simulink model "SLtest"  (R2024b)
settings: Solver=VariableStepAuto  StartTime=0.0  StopTime=10.0  RelTol=1e-3
settings Model: Creator=lazar  LastModifiedBy=lazar

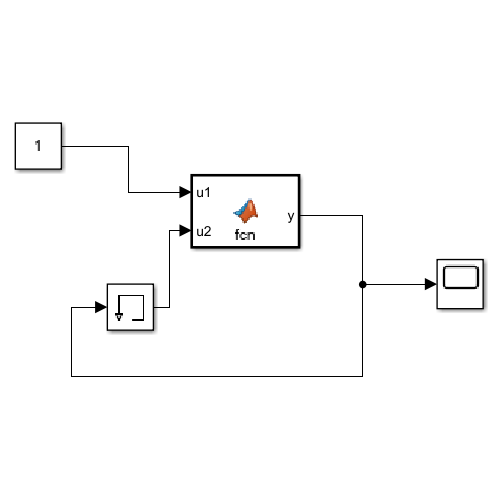
[thumbnail: Simulink's stored preview of the top-level diagram]
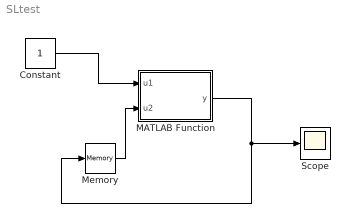
== system SLtest ==
  Constant : Constant
  MATLAB Function : MATLAB Function  TreatAsAtomicUnit=on
  Memory : Memory  InitialCondition=1
  Scope : Scope
  wires:
  Constant/1 -> MATLAB Function/1(u1)
  MATLAB Function/1(y) -> Scope/1, Memory/1
  Memory/1 -> MATLAB Function/2(u2)

== matlab function SLtest/MATLAB Function ==
  data: u1 input; y output; u2 input
function y = fcn(u1, u2)
    y = u1 + u2;  % Function adds two inputs
end
